simulink model "single_camera_xy_tracking_base_kf_fixed"  (R2025b)
settings: Solver=FixedStepDiscrete  StartTime=0  StopTime=T_end  FixedStep=Ts  RelTol=1e-3
InitFcn:
  | % 获取当前.slx模型所在文件夹
  | model_path = fileparts(which(gcs));
  | % 向上跳转、拼接目标函数所在文件夹（根据你的目录调整）
  | func_folder = fullfile(model_path,'..', 'config');
  | % 添加到搜索路径
  | addpath(func_folder);
  | % 执行初始化函数
  | init_single_camera_xy_tracking;
values from neighbouring files (symbols this model uses):
  a_xy_max = 2.0    (= 2)    [init_single_camera_xy_tracking.m]    (also in init_single_camera_xy_tracking_5dof.m; init_single_camera_xy_tracking_base_cv_kf.m; init_single_camera_xy_tracking_cv_ekf.m)
  adapt_max = 0.0    (= 0)    [init_single_camera_xy_tracking.m]    (also in init_single_camera_xy_tracking_5dof.m)
  camera_velocity_feedback_timeout_sec = 0.5    [init_single_camera_xy_tracking.m]    (also in init_single_camera_xy_tracking_5dof.m)
  controller_enable = true    [init_single_camera_xy_tracking.m]    (also in init_single_camera_xy_tracking_5dof.m; init_single_camera_xy_tracking_base_cv_kf.m; init_single_camera_xy_tracking_cv_ekf.m)
  cx = 1000    [init_single_camera_xy_tracking.m]    (also in init_single_camera_xy_tracking_5dof.m; init_single_camera_xy_tracking_base_cv_kf.m; init_single_camera_xy_tracking_cv_ekf.m)
  cy = 592    [init_single_camera_xy_tracking.m]    (also in init_single_camera_xy_tracking_5dof.m; init_single_camera_xy_tracking_base_cv_kf.m; init_single_camera_xy_tracking_cv_ekf.m)
  ekf_gate_threshold = 5.991    [init_single_camera_xy_tracking.m]    (also in init_single_camera_xy_tracking_5dof.m; init_single_camera_xy_tracking_cv_ekf.m)
  ekf_reset_timeout_sec = 0.50    (= 0.5)    [init_single_camera_xy_tracking.m]    (also in init_single_camera_xy_tracking_5dof.m; init_single_camera_xy_tracking_cv_ekf.m)
  enable_adaptation = false    [init_single_camera_xy_tracking_5dof.m]
  enable_ekf_feedforward = true    [init_single_camera_xy_tracking.m]    (also in init_single_camera_xy_tracking_5dof.m; init_single_camera_xy_tracking_base_cv_kf.m; init_single_camera_xy_tracking_cv_ekf.m)
  enable_proportional = true    [init_single_camera_xy_tracking.m]    (also in init_single_camera_xy_tracking_5dof.m; init_single_camera_xy_tracking_base_cv_kf.m; init_single_camera_xy_tracking_cv_ekf.m)
  fx = 2057    [init_single_camera_xy_tracking.m]    (also in init_single_camera_xy_tracking_5dof.m; init_single_camera_xy_tracking_base_cv_kf.m; init_single_camera_xy_tracking_cv_ekf.m)
  fy = 2054    [init_single_camera_xy_tracking.m]    (also in init_single_camera_xy_tracking_5dof.m; init_single_camera_xy_tracking_base_cv_kf.m; init_single_camera_xy_tracking_cv_ekf.m)
  gamma_adapt = 0.0    (= 0)    [init_single_camera_xy_tracking.m]    (also in init_single_camera_xy_tracking_5dof.m)
  joint_state_timeout_sec = 0.10    (= 0.1)    [init_single_camera_xy_tracking.m]    (also in init_single_camera_xy_tracking_5dof.m; init_single_camera_xy_tracking_base_cv_kf.m; init_single_camera_xy_tracking_cv_ekf.m)
  k_ff = 0.5    [init_single_camera_xy_tracking.m]    (also in init_single_camera_xy_tracking_5dof.m; init_single_camera_xy_tracking_base_cv_kf.m; init_single_camera_xy_tracking_cv_ekf.m)
  Kpx = 1.0    (= 1)    [init_single_camera_xy_tracking.m]    (also in init_single_camera_xy_tracking_5dof.m; init_single_camera_xy_tracking_base_cv_kf.m; init_single_camera_xy_tracking_cv_ekf.m)
  Kpy = 1.0    (= 1)    [init_single_camera_xy_tracking.m]    (also in init_single_camera_xy_tracking_5dof.m; init_single_camera_xy_tracking_base_cv_kf.m; init_single_camera_xy_tracking_cv_ekf.m)
  P0 = diag([0.05^2, 0.05^2, 0.20^2, 0.20^2, 0.50^2, 0.50^2])    [init_single_camera_xy_tracking.m]    (also in init_single_camera_xy_tracking_5dof.m = diag([.05 .05 .2 .2 .5 .5].^2); init_single_camera_xy_tracking_base_cv_kf.m = diag([.05 .05 .20 .20].^2); init_single_camera_xy_tracking_cv_ekf.m = diag([.05 .05 .20 .20].^2))
  Q_ekf = diag([1e-12, 1e-12, 1e-12, 1e-12, 1e-4, 1e-4])    [init_single_camera_xy_tracking.m]    (also in init_single_camera_xy_tracking_5dof.m = diag([1e-12 1e-12 1e-12 1e-12 1e-4 1e-4]); init_single_camera_xy_tracking_cv_ekf.m = sigma_acc_cv^2*[      Ts^4/4 0 Ts^3/2 0;      0 Ts^4/4 0 Ts^)
  R_ekf = diag([1e-8, 1e-8])    [init_single_camera_xy_tracking.m]    (also in init_single_camera_xy_tracking_5dof.m = diag([1e-8 1e-8]); init_single_camera_xy_tracking_cv_ekf.m = diag([1e-8 1e-8]))
  sigma_adapt = 0.0    (= 0)    [init_single_camera_xy_tracking.m]    (also in init_single_camera_xy_tracking_5dof.m)
  target_timeout_sec = 0.20    (= 0.2)    [init_single_camera_xy_tracking.m]    (also in init_single_camera_xy_tracking_5dof.m; init_single_camera_xy_tracking_base_cv_kf.m; init_single_camera_xy_tracking_cv_ekf.m)
  Ts = 0.01    [init_single_camera_xy_tracking.m]    (also in init_single_camera_xy_tracking_5dof.m; init_single_camera_xy_tracking_base_cv_kf.m; init_single_camera_xy_tracking_cv_ekf.m)
  v_xy_max = 2.0    (= 2)    [init_single_camera_xy_tracking.m]    (also in init_single_camera_xy_tracking_5dof.m; init_single_camera_xy_tracking_base_cv_kf.m; init_single_camera_xy_tracking_cv_ekf.m)
  Z_hat = 1    [init_single_camera_xy_tracking.m]    (also in init_single_camera_xy_tracking_5dof.m; init_single_camera_xy_tracking_base_cv_kf.m; init_single_camera_xy_tracking_cv_ekf.m)
undefined symbols (not defined in the file or in its folder): data, data_SL_Info
libraries: ros2lib x4, robotmaniplib x3
Description:
  | Fixed-focus monocular XY target tracking. Outputs camera-frame [vx vy 0 0 0 0]; robot kinematics remain external.
settings Model: Creator=ASUS  LastModifiedBy=harry
settings DataIOCC: SignalLogging=off

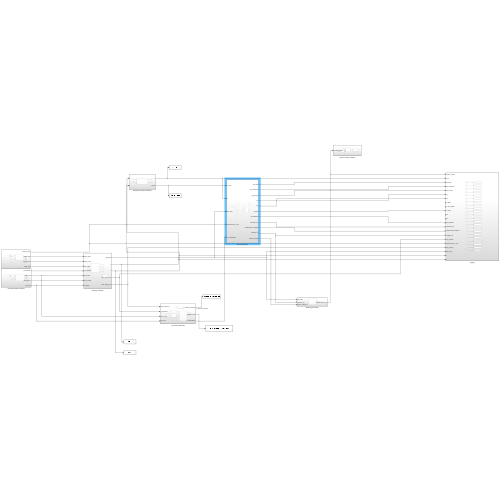
[thumbnail: Simulink's stored preview of the top-level diagram]
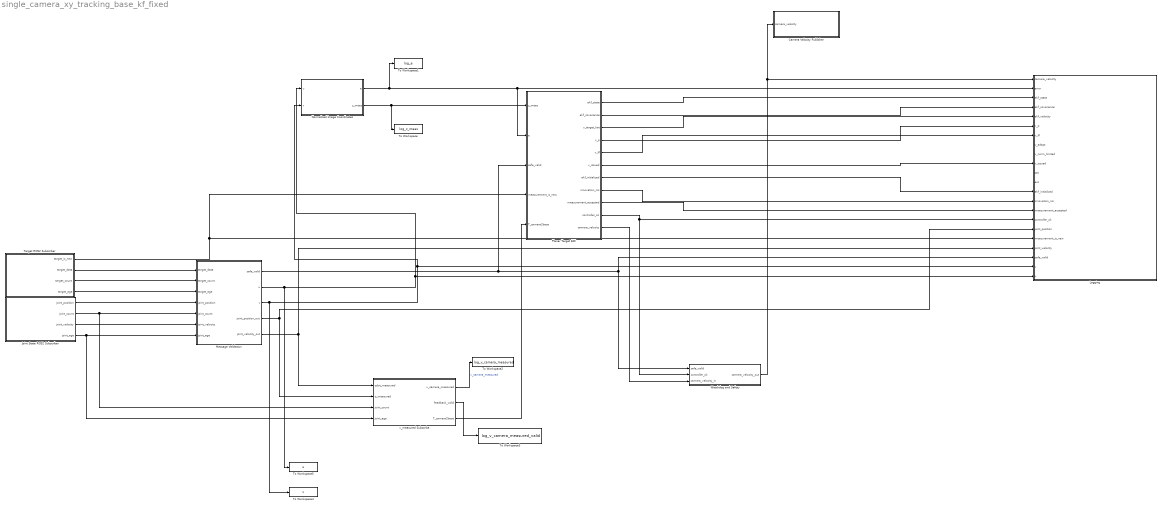
== system single_camera_xy_tracking_base_kf_fixed ==
  Camera Velocity Publisher : Subsystem
  Joint State ROS2 Subscriber : Subsystem
  Logging : Subsystem
  Message Validation : Subsystem
  Normalized Image Coordinates : Subsystem
  Planar Target EKF : Subsystem
  Target ROS2 Subscriber : Subsystem
  To Workspace : ToWorkspace  VariableName=log_z_meas  SaveFormat=Timeseries  SampleTime=-1
  To Workspace1 : ToWorkspace  VariableName=log_e  SaveFormat=Timeseries  SampleTime=-1
  To Workspace2 : ToWorkspace  VariableName=log_v_camera_measured  SaveFormat=Timeseries  SampleTime=-1
  To Workspace3 : ToWorkspace  VariableName=log_v_camera_measured_valid  SaveFormat=Timeseries  SampleTime=-1
  To Workspace4 : ToWorkspace  VariableName=v  SaveFormat=Timeseries  SampleTime=-1
  To Workspace5 : ToWorkspace  VariableName=u  SaveFormat=Timeseries  SampleTime=-1
  Watchdog and Safety : Subsystem
  v_measured Subscribe : Subsystem
  wires:
  Target ROS2 Subscriber/4(target_age) -> Message Validation/3(target_age)
  Target ROS2 Subscriber/2(target_data) -> Message Validation/1(target_data)
  Target ROS2 Subscriber/3(target_count) -> Message Validation/2(target_count)
  Planar Target EKF/3(v_target_hat) -> Logging/5(ekf_velocity)
  Message Validation/2(u) -> Normalized Image Coordinates/1(u), Logging/22(u), To Workspace5/1
  Planar Target EKF/10(controller_ok) -> Watchdog and Safety/2(controller_ok), Logging/16(controller_ok)
  Joint State ROS2 Subscriber/4(joint_age) -> v_measured Subscribe/4(joint_age), Message Validation/7(joint_age)
  Joint State ROS2 Subscriber/2(joint_count) -> v_measured Subscribe/3(joint_count), Message Validation/5(joint_count)
  Joint State ROS2 Subscriber/1(joint_position) -> Message Validation/4(joint_position)
  Joint State ROS2 Subscriber/3(joint_velocity) -> Message Validation/6(joint_velocity)
  Message Validation/1(safe_valid) -> Logging/20(safe_valid), Watchdog and Safety/1(safe_valid), Planar Target EKF/3(safe_valid)
  Message Validation/3(v) -> To Workspace4/1, Normalized Image Coordinates/2(v), Logging/21(v)
  Message Validation/4(joint_position_out) -> v_measured Subscribe/2(q_measured), Logging/17(joint_position)
  Message Validation/5(joint_velocity_out) -> v_measured Subscribe/1(qdot_measured), Logging/19(joint_velocity)
  Normalized Image Coordinates/1(e) -> To Workspace1/1, Logging/2(error), Planar Target EKF/2(e)
  Normalized Image Coordinates/2(z_meas) -> To Workspace/1, Planar Target EKF/1(z_meas)
  Planar Target EKF/1(ekf_state) -> Logging/3(ekf_state)
  Planar Target EKF/2(ekf_covariance) -> Logging/4(ekf_covariance)
  Planar Target EKF/9(measurement_accepted) -> Logging/15(measurement_accepted)
  Planar Target EKF/7(ekf_initialized) -> Logging/13(ekf_initialized)
  Planar Target EKF/8(innovation_nis) -> Logging/14(innovation_nis)
  Planar Target EKF/4(v_p) -> Logging/6(v_p)
  Planar Target EKF/5(v_ff) -> Logging/7(v_ff)
  Planar Target EKF/6(v_issued) -> Logging/10(v_issued)
  Planar Target EKF/11(camera_velocity) -> Watchdog and Safety/3(camera_velocity_in)
  Watchdog and Safety/1(camera_velocity_out) -> Camera Velocity Publisher/1(camera_velocity), Logging/1(camera_velocity)
  Target ROS2 Subscriber/1(target_is_new) -> Planar Target EKF/4(measurement_is_new), Logging/18(measurement_is_new)
  v_measured Subscribe/1(v_camera_measured) -> To Workspace2/1  "v_camera_measured"
  v_measured Subscribe/2(feedback_valid) -> To Workspace3/1
  v_measured Subscribe/3(T_camera2base) -> Planar Target EKF/5(T_camera2base)

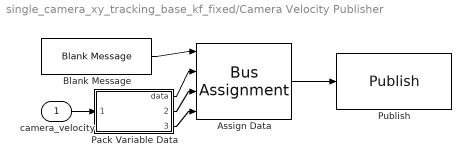
== system single_camera_xy_tracking_base_kf_fixed/Camera Velocity Publisher ==
  camera_velocity : Inport
  Assign Data : BusAssignment  AssignedSignals=data,data_SL_Info.CurrentLength,data_SL_Info.ReceivedLength
  Blank Message : ros2lib/Blank Message  messageClass=Message  entityType=std_msgs/Float64MultiArray  messageType=std_msgs/Float64MultiArray  SampleTime=Ts
  Pack Variable Data : MATLAB Function  TreatAsAtomicUnit=on
  Publish : ros2lib/Publish  topicSource=Select from ROS network  topic=/simulink/camera_velocity  messageType=std_msgs/Float64MultiArray  QOSHistory=Keep last  QOSDepth=1  QOSReliability=Reliable  QOSDurability=Volatile  QOSDeadline=Inf  QOSLifespan=Inf  QOSLiveliness=Automatic  QOSLeaseDuration=Inf  QOSAvoidROSNamespaceConventions=off
  wires:
  Blank Message/1 -> Assign Data/1
  Assign Data/1 -> Publish/1
  camera_velocity/1 -> Pack Variable Data/1(camera_velocity)
  Pack Variable Data/1(data) -> Assign Data/2
  Pack Variable Data/2(current_length) -> Assign Data/3
  Pack Variable Data/3(received_length) -> Assign Data/4

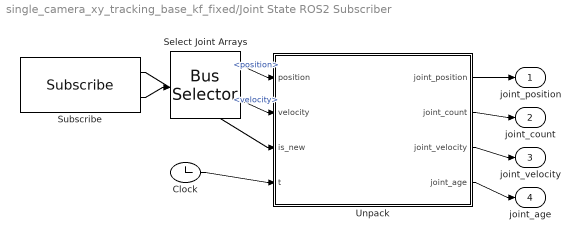
== system single_camera_xy_tracking_base_kf_fixed/Joint State ROS2 Subscriber ==
  Clock : Clock
  Select Joint Arrays : BusSelector  OutputSignals=position,velocity
  Subscribe : ros2lib/Subscribe  topicSource=Select from ROS network  topic=/franka/joint_states  messageType=sensor_msgs/JointState  sampleTime=Ts  QOSHistory=Keep last  QOSDepth=1  QOSReliability=Best effort  QOSDurability=Volatile  QOSDeadline=Inf  QOSLifespan=Inf  QOSLiveliness=Automatic  QOSLeaseDuration=Inf  QOSAvoidROSNamespaceConventions=off
  Unpack : MATLAB Function  TreatAsAtomicUnit=on
  joint_position : Outport
  joint_count : Outport  Port=2
  joint_velocity : Outport  Port=3
  joint_age : Outport  Port=4
  wires:
  Unpack/1(joint_position) -> joint_position/1
  Unpack/2(joint_count) -> joint_count/1
  Unpack/3(joint_velocity) -> joint_velocity/1
  Unpack/4(joint_age) -> joint_age/1
  Select Joint Arrays/1 -> Unpack/1(position)  "<position>"
  Select Joint Arrays/2 -> Unpack/2(velocity)  "<velocity>"
  Clock/1 -> Unpack/4(t)
  Subscribe/2 -> Select Joint Arrays/1
  Subscribe/1 -> Unpack/3(is_new)

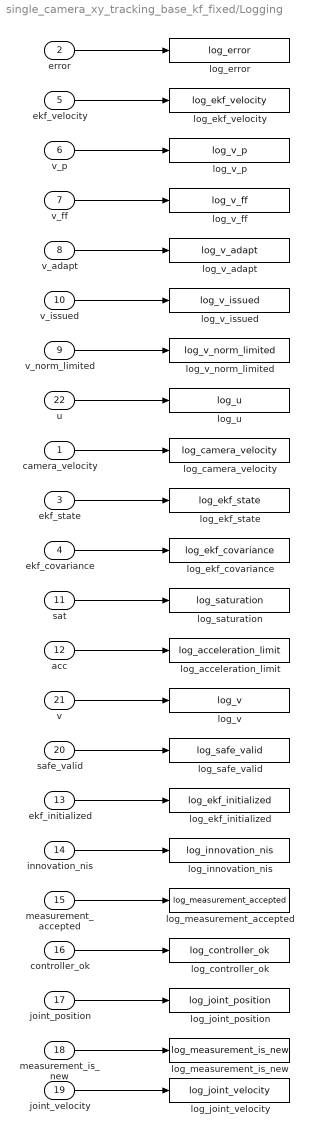
== system single_camera_xy_tracking_base_kf_fixed/Logging ==
  camera_velocity : Inport
  error : Inport  Port=2
  ekf_state : Inport  Port=3
  ekf_covariance : Inport  Port=4
  ekf_velocity : Inport  Port=5
  v_p : Inport  Port=6
  v_ff : Inport  Port=7
  v_adapt : Inport  Port=8
  v_norm_limited : Inport  Port=9
  v_issued : Inport  Port=10
  sat : Inport  Port=11
  acc : Inport  Port=12
  ekf_initialized : Inport  Port=13
  innovation_nis : Inport  Port=14
  measurement_accepted : Inport  Port=15
  controller_ok : Inport  Port=16
  joint_position : Inport  Port=17
  measurement_is_new : Inport  Port=18
  joint_velocity : Inport  Port=19
  safe_valid : Inport  Port=20
  v : Inport  Port=21
  u : Inport  Port=22
  log_acceleration_limit : ToWorkspace  VariableName=log_acceleration_limit  SaveFormat=Structure With Time  SampleTime=-1
  log_camera_velocity : ToWorkspace  VariableName=log_camera_velocity  SaveFormat=Structure With Time  SampleTime=-1
  log_controller_ok : ToWorkspace  VariableName=log_controller_ok  SaveFormat=Structure With Time  SampleTime=-1
  log_ekf_covariance : ToWorkspace  VariableName=log_ekf_covariance  SaveFormat=Structure With Time  SampleTime=-1
  log_ekf_initialized : ToWorkspace  VariableName=log_ekf_initialized  SaveFormat=Structure With Time  SampleTime=-1
  log_ekf_state : ToWorkspace  VariableName=log_ekf_state  SaveFormat=Structure With Time  SampleTime=-1
  log_ekf_velocity : ToWorkspace  VariableName=log_ekf_velocity  SaveFormat=Structure With Time  SampleTime=-1
  log_error : ToWorkspace  VariableName=log_error  SaveFormat=Structure With Time  SampleTime=-1
  log_innovation_nis : ToWorkspace  VariableName=log_innovation_nis  SaveFormat=Structure With Time  SampleTime=-1
  log_joint_position : ToWorkspace  VariableName=log_joint_position  SaveFormat=Structure With Time  SampleTime=-1
  log_joint_velocity : ToWorkspace  VariableName=log_joint_velocity  SaveFormat=Structure With Time  SampleTime=-1
  log_measurement_accepted : ToWorkspace  VariableName=log_measurement_accepted  SaveFormat=Structure With Time  SampleTime=-1
  log_measurement_is_new : ToWorkspace  VariableName=log_measurement_is_new  SaveFormat=Structure With Time  SampleTime=-1
  log_safe_valid : ToWorkspace  VariableName=log_safe_valid  SaveFormat=Structure With Time  SampleTime=-1
  log_saturation : ToWorkspace  VariableName=log_saturation  SaveFormat=Structure With Time  SampleTime=-1
  log_u : ToWorkspace  VariableName=log_u  SaveFormat=Structure With Time  SampleTime=-1
  log_v : ToWorkspace  VariableName=log_v  SaveFormat=Structure With Time  SampleTime=-1
  log_v_adapt : ToWorkspace  VariableName=log_v_adapt  SaveFormat=Structure With Time  SampleTime=-1
  log_v_ff : ToWorkspace  VariableName=log_v_ff  SaveFormat=Structure With Time  SampleTime=-1
  log_v_issued : ToWorkspace  VariableName=log_v_issued  SaveFormat=Structure With Time  SampleTime=-1
  log_v_norm_limited : ToWorkspace  VariableName=log_v_norm_limited  SaveFormat=Structure With Time  SampleTime=-1
  log_v_p : ToWorkspace  VariableName=log_v_p  SaveFormat=Structure With Time  SampleTime=-1
  wires:
  error/1 -> log_error/1
  ekf_velocity/1 -> log_ekf_velocity/1
  v_p/1 -> log_v_p/1
  v_ff/1 -> log_v_ff/1
  v_adapt/1 -> log_v_adapt/1
  v_issued/1 -> log_v_issued/1
  u/1 -> log_u/1
  camera_velocity/1 -> log_camera_velocity/1
  ekf_state/1 -> log_ekf_state/1
  ekf_covariance/1 -> log_ekf_covariance/1
  sat/1 -> log_saturation/1
  acc/1 -> log_acceleration_limit/1
  v/1 -> log_v/1
  safe_valid/1 -> log_safe_valid/1
  ekf_initialized/1 -> log_ekf_initialized/1
  innovation_nis/1 -> log_innovation_nis/1
  measurement_accepted/1 -> log_measurement_accepted/1
  controller_ok/1 -> log_controller_ok/1
  joint_position/1 -> log_joint_position/1
  joint_velocity/1 -> log_joint_velocity/1
  measurement_is_new/1 -> log_measurement_is_new/1
  v_norm_limited/1 -> log_v_norm_limited/1

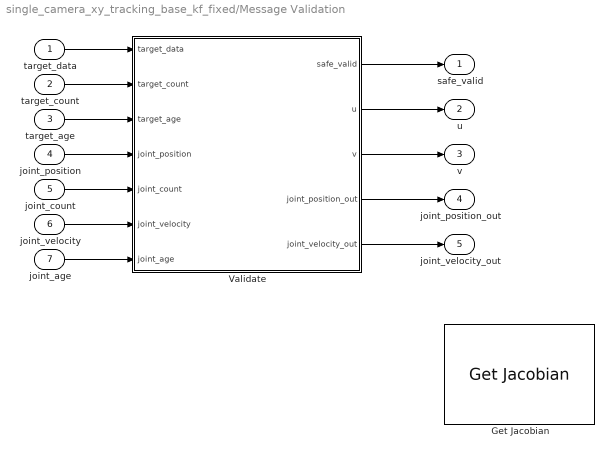
== system single_camera_xy_tracking_base_kf_fixed/Message Validation ==
  target_data : Inport
  target_count : Inport  Port=2
  target_age : Inport  Port=3
  joint_position : Inport  Port=4
  joint_count : Inport  Port=5
  joint_velocity : Inport  Port=6
  joint_age : Inport  Port=7
  Get Jacobian : robotmaniplib/Get Jacobian  RigidBodyTree=twoJointRigidBodyTree  EndEffector=tool  SimulateUsing=Interpreted execution
  Validate : MATLAB Function  TreatAsAtomicUnit=on
  safe_valid : Outport
  u : Outport  Port=2
  v : Outport  Port=3
  joint_position_out : Outport  Port=4
  joint_velocity_out : Outport  Port=5
  wires:
  Validate/1(safe_valid) -> safe_valid/1
  Validate/2(u) -> u/1
  Validate/3(v) -> v/1
  Validate/4(joint_position_out) -> joint_position_out/1
  Validate/5(joint_velocity_out) -> joint_velocity_out/1
  target_data/1 -> Validate/1(target_data)
  target_count/1 -> Validate/2(target_count)
  target_age/1 -> Validate/3(target_age)
  joint_position/1 -> Validate/4(joint_position)
  joint_count/1 -> Validate/5(joint_count)
  joint_velocity/1 -> Validate/6(joint_velocity)
  joint_age/1 -> Validate/7(joint_age)

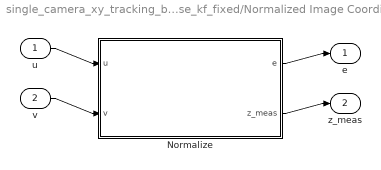
== system single_camera_xy_tracking_base_kf_fixed/Normalized Image Coordinates ==
  u : Inport
  v : Inport  Port=2
  Normalize : MATLAB Function  TreatAsAtomicUnit=on
  e : Outport
  z_meas : Outport  Port=2
  wires:
  u/1 -> Normalize/1(u)
  v/1 -> Normalize/2(v)
  Normalize/1(e) -> e/1
  Normalize/2(z_meas) -> z_meas/1

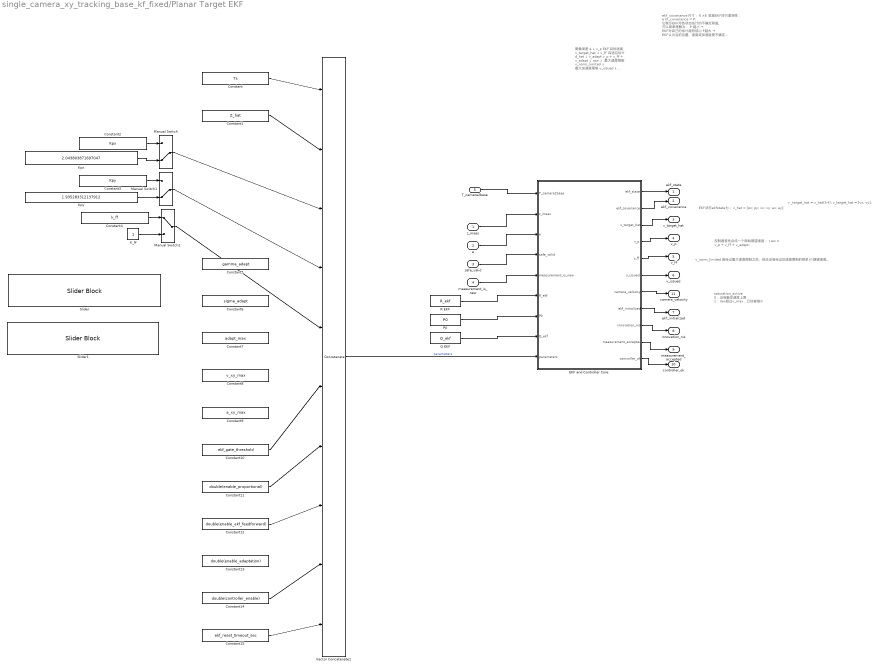
== system single_camera_xy_tracking_base_kf_fixed/Planar Target EKF ==
  note: saturation_active
      | 0：没有触发速度上限
      | 1：raw超过v_max，已经被缩小
  note: ekf_covariance
      | 尺寸：
      | 6 ×6
      | 就是EKF协方差矩阵：
      | e kf_covariance = P;
      | 它表示EKF对各状态估计的不确定程度。
      | 可以简单理解为：
      | P 越小
      | → EKF对自己的估计越有信心
      |
      | P越大
      | → EKF认为当前位置、速度或加速度更不确定
      | 重点可以观察：
      | d iag(P)
      | 也就是：
      | 位 置方差
      | 速度方差
      | 加速度方差
  note: 图像误差 e
      |     ↓
      | v_p
      |
      | EKF目标速度 v_target_hat
      |     ↓
      | v_ff
      |
      | 自适应估计 d_hat
      |     ↓
      | v_adapt
      |
      | v_p + v_ff + v_adapt
      |     ↓
      | raw
      |     ↓ 最大速度限制
      | v_norm_limited
      |     ↓ 最大加速度限制
      | v_issued
      |     ↓ 扩展为6维
      | camera_velocity
  note: EKF状态ekfstate为： x_hat = [px; py; vx; vy; ax; ay];
  note: v _target_hat = x_hat(3:4); v_target_hat = [vx; vy];
  note: 控制器首先合成一个原始期望速度：
      | r aw = v_p + v_ff + v_adapt;
  note: v_norm_limited 是经过最大速度限制之后、但还没有经过加速度限制的相机XY期望速度。
  z_meas : Inport
  e : Inport  Port=2
  safe_valid : Inport  Port=3
  measurement_is_new : Inport  Port=4
  T_camera2base : Inport  Port=5
  Constant : Constant  Value=Ts
  Constant1 : Constant  Value=Z_hat
  Constant10 : Constant  Value=ekf_gate_threshold
  Constant11 : Constant  Value=double(enable_proportional)
  Constant12 : Constant  Value=double(enable_ekf_feedforward)
  Constant13 : Constant  Value=double(enable_adaptation)
  Constant14 : Constant  Value=double(controller_enable)
  Constant15 : Constant  Value=ekf_reset_timeout_sec
  Constant2 : Constant  Value=Kpx
  Constant3 : Constant  Value=Kpy
  Constant4 : Constant  Value=k_ff
  Constant5 : Constant  Value=gamma_adapt
  Constant6 : Constant  Value=sigma_adapt
  Constant7 : Constant  Value=adapt_max
  Constant8 : Constant  Value=v_xy_max
  Constant9 : Constant  Value=a_xy_max
  EKF and Controller Core : MATLAB Function  TreatAsAtomicUnit=on
  K_ff : Constant
  Kpx : Constant  Value=2.043803871697047
  Kpy : Constant  Value=1.935283312137912
  Manual Switch : ManualSwitch  CurrentSetting=0
  Manual Switch1 : ManualSwitch  CurrentSetting=0
  Manual Switch2 : ManualSwitch
  P0 : Constant  Value=P0
  Q EKF : Constant  Value=Q_ekf
  R EKF : Constant  Value=R_ekf
  Slider : SliderBlock  ScaleMax=10
  Slider1 : SliderBlock  ScaleMax=10
  Vector Concatenate1 : Concatenate  NumInputs=10
  ekf_state : Outport
  ekf_covariance : Outport  Port=2
  v_target_hat : Outport  Port=3
  v_p : Outport  Port=4
  v_ff : Outport  Port=5
  v_issued : Outport  Port=6
  ekf_initialized : Outport  Port=7
  innovation_nis : Outport  Port=8
  measurement_accepted : Outport  Port=9
  controller_ok : Outport  Port=10
  camera_velocity : Outport  Port=11
  wires:
  EKF and Controller Core/1(ekf_state) -> ekf_state/1
  EKF and Controller Core/2(ekf_covariance) -> ekf_covariance/1
  EKF and Controller Core/3(v_target_hat) -> v_target_hat/1
  EKF and Controller Core/4(v_p) -> v_p/1
  EKF and Controller Core/5(v_ff) -> v_ff/1
  EKF and Controller Core/6(v_issued) -> v_issued/1
  EKF and Controller Core/7(camera_velocity) -> camera_velocity/1
  EKF and Controller Core/8(ekf_initialized) -> ekf_initialized/1
  EKF and Controller Core/9(innovation_nis) -> innovation_nis/1
  EKF and Controller Core/10(measurement_accepted) -> measurement_accepted/1
  EKF and Controller Core/11(controller_ok) -> controller_ok/1
  z_meas/1 -> EKF and Controller Core/2(z_meas)
  e/1 -> EKF and Controller Core/3(e)
  safe_valid/1 -> EKF and Controller Core/4(safe_valid)
  measurement_is_new/1 -> EKF and Controller Core/5(measurement_is_new)
  Vector Concatenate1/1 -> EKF and Controller Core/9(parameters)  "parameters"
  P0/1 -> EKF and Controller Core/7(P0)
  Q EKF/1 -> EKF and Controller Core/8(Q_ekf)
  R EKF/1 -> EKF and Controller Core/6(R_ekf)
  Constant/1 -> Vector Concatenate1/1
  Constant1/1 -> Vector Concatenate1/2
  Constant10/1 -> Vector Concatenate1/6
  Constant11/1 -> Vector Concatenate1/7
  Constant12/1 -> Vector Concatenate1/8
  Constant14/1 -> Vector Concatenate1/9
  Constant15/1 -> Vector Concatenate1/10
  T_camera2base/1 -> EKF and Controller Core/1(T_camera2base)
  Constant2/1 -> Manual Switch/1
  Manual Switch/1 -> Vector Concatenate1/3
  Kpx/1 -> Manual Switch/2
  Kpy/1 -> Manual Switch1/2
  Constant3/1 -> Manual Switch1/1
  Manual Switch1/1 -> Vector Concatenate1/4
  Constant4/1 -> Manual Switch2/1
  Manual Switch2/1 -> Vector Concatenate1/5
  K_ff/1 -> Manual Switch2/2

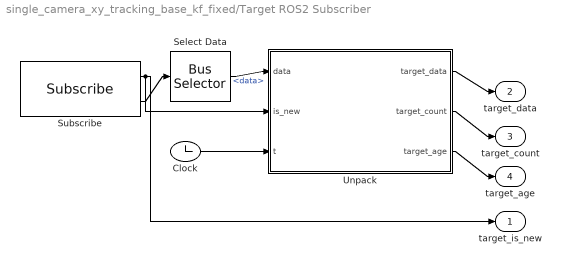
== system single_camera_xy_tracking_base_kf_fixed/Target ROS2 Subscriber ==
  Clock : Clock
  Select Data : BusSelector  OutputSignals=data
  Subscribe : ros2lib/Subscribe  topicSource=Select from ROS network  topic=/apriltag_detector/target_position  messageType=std_msgs/Float64MultiArray  sampleTime=Ts  QOSHistory=Keep last  QOSDepth=1  QOSReliability=Best effort  QOSDurability=Volatile  QOSDeadline=Inf  QOSLifespan=Inf  QOSLiveliness=Automatic  QOSLeaseDuration=Inf  QOSAvoidROSNamespaceConventions=off
  Unpack : MATLAB Function  TreatAsAtomicUnit=on
  target_is_new : Outport
  target_data : Outport  Port=2
  target_count : Outport  Port=3
  target_age : Outport  Port=4
  wires:
  Unpack/1(target_data) -> target_data/1
  Unpack/2(target_count) -> target_count/1
  Unpack/3(target_age) -> target_age/1
  Select Data/1 -> Unpack/1(data)  "<data>"
  Clock/1 -> Unpack/3(t)
  Subscribe/2 -> Select Data/1
  Subscribe/1 -> Unpack/2(is_new), target_is_new/1

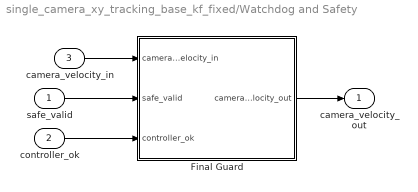
== system single_camera_xy_tracking_base_kf_fixed/Watchdog and Safety ==
  safe_valid : Inport
  controller_ok : Inport  Port=2
  camera_velocity_in : Inport  Port=3
  Final Guard : MATLAB Function  TreatAsAtomicUnit=on
  camera_velocity_out : Outport
  wires:
  camera_velocity_in/1 -> Final Guard/1(camera_velocity_in)
  safe_valid/1 -> Final Guard/2(safe_valid)
  controller_ok/1 -> Final Guard/3(controller_ok)
  Final Guard/1(camera_velocity_out) -> camera_velocity_out/1

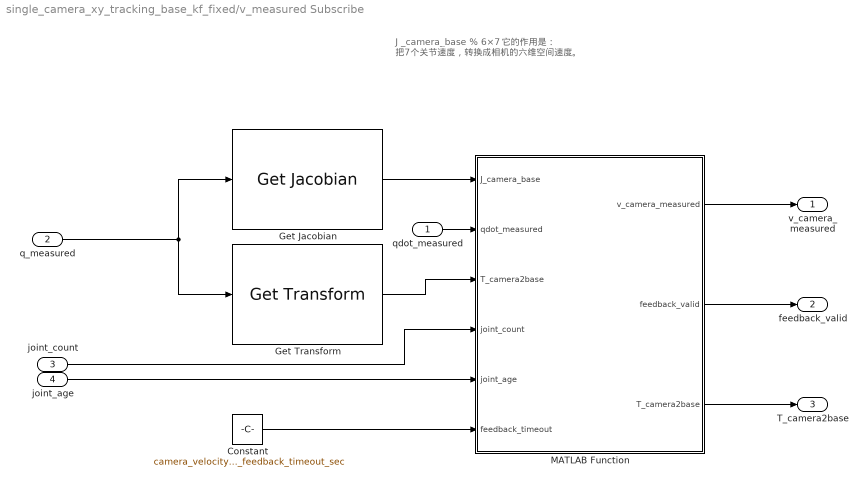
== system single_camera_xy_tracking_base_kf_fixed/v_measured Subscribe ==
  note: J _camera_base % 6×7
      | 它的作用是：
      | 把7个关节速度，转换成相机的六维空间速度。
  qdot_measured : Inport
  q_measured : Inport  Port=2
  joint_count : Inport  Port=3
  joint_age : Inport  Port=4
  Constant : Constant  Value=camera_velocity_feedback_timeout_sec
  Get Jacobian : robotmaniplib/Get Jacobian  RigidBodyTree=fr3_camera_robot  EndEffector=camera_link  SimulateUsing=Interpreted execution
  Get Transform : robotmaniplib/Get Transform  RigidBodyTree=fr3_camera_robot  SourceBody=camera_link  TargetBody=base  SimulateUsing=Interpreted execution
  MATLAB Function : MATLAB Function  TreatAsAtomicUnit=on
  v_camera_measured : Outport
  feedback_valid : Outport  Port=2
  T_camera2base : Outport  Port=3
  wires:
  q_measured/1 -> Get Transform/1, Get Jacobian/1
  qdot_measured/1 -> MATLAB Function/2(qdot_measured)
  Get Jacobian/1 -> MATLAB Function/1(J_camera_base)
  Get Transform/1 -> MATLAB Function/3("T_camera2base ")
  joint_count/1 -> MATLAB Function/4(joint_count)
  joint_age/1 -> MATLAB Function/5(joint_age)
  Constant/1 -> MATLAB Function/6(feedback_timeout)
  MATLAB Function/1(v_camera_measured) -> v_camera_measured/1
  MATLAB Function/2(feedback_valid) -> feedback_valid/1
  MATLAB Function/3(T_camera2base) -> T_camera2base/1

== matlab function single_camera_xy_tracking_base_kf_fixed/Planar Target EKF/EKF and Controller Core ==
  data: T_camera2base input; z_meas input size=[2 1]; ekf_state output size=[6 1]; e input size=[2 1]; safe_valid input size=1; measurement_is_new input; R_ekf input size=[2 2]; P0 input size=[6 6]; Q_ekf input size=[6 6]; parameters input size=[16 1]; ekf_covariance output size=[6 6]; v_target_hat output size=[2 1]; v_p output size=[2 1]; v_ff output size=[2 1]; v_issued output size=[2 1]; camera_velocity output size=[6 1]; ekf_initialized output size=1; innovation_nis output size=1; measurement_accepted output size=1; controller_ok output size=1
function [ ...
    ekf_state, ...
    ekf_covariance, ...
    v_target_hat, ...
    v_p, ...
    v_ff, ...
    v_issued, ...
    camera_velocity, ...
    ekf_initialized, ...
    innovation_nis, ...
    measurement_accepted, ...
    controller_ok] = fcn( ...
    T_camera2base, ...
    z_meas, ...
    e, ...
    safe_valid, ...
    measurement_is_new, ...
    R_ekf, ...
    P0, ...
    Q_ekf, ...
    parameters)
%#codegen
%
% Base坐标系目标状态估计与相机XY速度控制器。
%
% ==================== 坐标系定义 ====================
%
% KF状态全部在机器人Base坐标系中：
%
% x_hat = [X_B; Y_B; Vx_B; Vy_B; Ax_B; Ay_B]
%
% z_meas为相机坐标系中的目标XY位置：
%
% z_meas = [X_C; Y_C]
%
% 根据固定深度Z_hat构造目标相机系三维位置：
%
% p_target_C = [X_C; Y_C; Z_hat]
%
% 再通过T_camera2base转换到机器人Base坐标系：
%
% p_target_B = R_BC*p_target_C + t_BC
%
% 控制器输出仍在相机坐标系：
%
% camera_velocity = [vx_C; vy_C; 0; 0; 0; 0]
%
% ==================== 输入矩阵要求 ====================
%
% T_camera2base：4×4，相机坐标系到Base坐标系的变换
%
%   p_B = T_camera2base*[p_C;1]
%
% R_ekf：2×2，相机系XY位置测量噪声协方差
% P0：6×6，Base系状态初始协方差
% Q_ekf：6×6，Base系过程噪声协方差
%
% ==================== parameters ====================
%
% parameters(1)  = Ts
% parameters(2)  = Z_hat
% parameters(3)  = Kpx
% parameters(4)  = Kpy
% parameters(5)  = k_ff
% parameters(6)  = NIS gate
% parameters(7)  = enable_p
% parameters(8)  = enable_ff
% parameters(9)  = controller_enable
% parameters(10) = reset_timeout


%% 1. 持久状态

persistent x_hat
persistent P
persistent e_hold
persistent invalid_time
persistent initialized


%% 2. 初始化

if isempty(initialized)

    x_hat = zeros(6,1);
    P = P0;

    e_hold = zeros(2,1);

    invalid_time = 0.0;
    initialized = false;
end


%% 3. 参数解析

Ts = parameters(1);
Z_hat = parameters(2);

Kpx = parameters(3);
Kpy = parameters(4);

k_ff = parameters(5);
gate = parameters(6);

enable_p = parameters(7) > 0.5;
enable_ff = parameters(8) > 0.5;

controller_enable = parameters(9) > 0.5;
reset_timeout = parameters(10);

safe_valid = safe_valid > 0.5;
measurement_is_new = measurement_is_new > 0.5;


%% 4. 默认输出

ekf_state = x_hat;
ekf_covariance = P;

% Base坐标系中的目标XY速度。
v_target_hat = zeros(2,1);

% 以下控制速度均在相机坐标系。
v_p = zeros(2,1);
v_ff = zeros(2,1);
v_issued = zeros(2,1);

camera_velocity = zeros(6,1);

ekf_initialized = initialized;

innovation_nis = NaN;
measurement_accepted = false;
controller_ok = false;


%% 5. 状态模型

% Base坐标系恒加速度模型：
%
% X(k+1)  = X(k)  + Ts*Vx(k) + 0.5*Ts^2*Ax(k)
% Y(k+1)  = Y(k)  + Ts*Vy(k) + 0.5*Ts^2*Ay(k)
% Vx(k+1) = Vx(k) + Ts*Ax(k)
% Vy(k+1) = Vy(k) + Ts*Ay(k)

F = [ ...
    1 0 Ts 0  0.5*Ts*Ts 0;
    0 1 0  Ts 0  0.5*Ts*Ts;
    0 0 1  0  Ts 0;
    0 0 0  1  0  Ts;
    0 0 0  0  1  0;
    0 0 0  0  0  1];

% 只测量Base坐标系目标XY位置。
H = [ ...
    1 0 0 0 0 0;
    0 1 0 0 0 0];

I6 = eye(6);


%% 6. 参数检查

parameter_ok = ...
    numel(parameters) >= 10 && ...
    isequal(size(P0),[6 6]) && ...
    isequal(size(Q_ekf),[6 6]) && ...
    isequal(size(R_ekf),[2 2]) && ...
    all(isfinite(parameters(:))) && ...
    all(isfinite(P0(:))) && ...
    all(isfinite(Q_ekf(:))) && ...
    all(isfinite(R_ekf(:))) && ...
    Ts > 0 && ...
    Z_hat > 0 && ...
    gate > 0 && ...
    reset_timeout >= Ts;

if ~parameter_ok

    x_hat = zeros(6,1);
    P = P0;

    e_hold = zeros(2,1);
    invalid_time = 0.0;
    initialized = false;

    ekf_state = x_hat;
    ekf_covariance = P;
    ekf_initialized = false;

    return
end


%% 7. 检查相机位姿

pose_matrix_ok = ...
    isequal(size(T_camera2base),[4 4]) && ...
    all(isfinite(T_camera2base(:)));

R_base_camera = eye(3);
t_base_camera = zeros(3,1);

pose_ok = false;

if pose_matrix_ok

    R_candidate = T_camera2base(1:3,1:3);
    t_candidate = T_camera2base(1:3,4);

    orthogonality_error = ...
        norm(R_candidate'*R_candidate - eye(3),'fro');

    determinant_error = ...
        abs(det(R_candidate) - 1.0);

    last_row_error = ...
        norm(T_camera2base(4,:) - [0 0 0 1]);

    pose_ok = ...
        orthogonality_error < 1e-3 && ...
        determinant_error < 1e-3 && ...
        last_row_error < 1e-6 && ...
        all(isfinite(t_candidate));

    if pose_ok
        R_base_camera = R_candidate;
        t_base_camera = t_candidate;
    end
end


%% 8. 检查视觉输入

vision_signal_ok = ...
    safe_valid && ...
    numel(z_meas) == 2 && ...
    numel(e) == 2 && ...
    all(isfinite(z_meas(:))) && ...
    all(isfinite(e(:)));


%% 9. 输入无效处理

if ~vision_signal_ok

    % 已初始化时继续执行纯预测。
    if initialized

        x_hat = F*x_hat;

        P = F*P*F' + Q_ekf;
        P = 0.5*(P + P');
    end

    invalid_time = invalid_time + Ts;

    % 没有有效目标时不继续使用旧图像误差。
    e_hold = zeros(2,1);

    state_ok = ...
        all(isfinite(x_hat(:))) && ...
        all(isfinite(P(:))) && ...
        all(diag(P) >= 0);

    if invalid_time >= reset_timeout || ~state_ok

        x_hat = zeros(6,1);
        P = P0;

        initialized = false;
    end

    ekf_state = x_hat;
    ekf_covariance = P;

    v_target_hat = x_hat(3:4);
    ekf_initialized = initialized;

    return
end

invalid_time = 0.0;


%% 10. 构造Base坐标系目标位置测量

measurement_available = ...
    measurement_is_new && ...
    pose_ok;

z_base = zeros(2,1);
R_measurement_base = R_ekf;

if measurement_available

    % 目标在相机坐标系中的三维位置。
    p_target_camera = [ ...
        z_meas(1);
        z_meas(2);
        Z_hat];

    % 转换到机器人Base坐标系。
    p_target_base = ...
        R_base_camera*p_target_camera + ...
        t_base_camera;

    % 当前滤波器只使用Base坐标系XY位置。
    z_base = p_target_base(1:2);

    % 将相机系XY测量噪声近似转换到Base系XY。
    %
    % 当前假设Z_hat没有额外测量噪声。
    measurement_rotation = ...
        R_base_camera(1:2,1:2);

    R_measurement_base = ...
        measurement_rotation*R_ekf* ...
        measurement_rotation';

    R_measurement_base = ...
        0.5*(R_measurement_base + ...
        R_measurement_base');

    measurement_available = ...
        all(isfinite(z_base(:))) && ...
        all(isfinite(R_measurement_base(:)));
end


%% 11. 更新最近一次图像误差

% 图像误差直接用于比例反馈。
% 它不受NIS是否接受Base位置测量的影响。

if measurement_is_new
    e_hold = reshape(e,2,1);
end


%% 12. 初始化滤波器

if ~initialized

    if ~measurement_available
        return
    end

    % 初始Base位置由当前目标测量给出。
    % 初始速度和加速度设为零。
    x_hat = [ ...
        z_base(1);
        z_base(2);
        0;
        0;
        0;
        0];

    P = P0;

    initialized = true;
    measurement_accepted = true;


%% 13. 状态预测与测量更新

else

    % 每个控制周期进行状态预测。
    x_pred = F*x_hat;

    P_pred = F*P*F' + Q_ekf;
    P_pred = 0.5*(P_pred + P_pred');

    % 默认采用预测结果。
    x_hat = x_pred;
    P = P_pred;

    if measurement_available

        % Base坐标系位置残差。
        innovation = ...
            z_base - H*x_pred;

        % 创新协方差。
        S = ...
            H*P_pred*H' + ...
            R_measurement_base;

        if all(isfinite(S(:))) && ...
                rcond(S) > 1e-12

            innovation_nis = ...
                innovation'*(S\innovation);

        else

            innovation_nis = inf;
        end

        % 通过NIS门限后进行测量更新。
        if isfinite(innovation_nis) && ...
                innovation_nis <= gate

            % 卡尔曼增益。
            K = ...
                (P_pred*H')/S;

            % 状态更新。
            x_hat = ...
                x_pred + K*innovation;

            % Joseph形式协方差更新。
            A = I6 - K*H;

            P = ...
                A*P_pred*A' + ...
                K*R_measurement_base*K';

            P = 0.5*(P + P');

            measurement_accepted = true;
        end
    end
end


%% 14. 滤波器状态检查

ekf_ok = ...
    all(isfinite(x_hat(:))) && ...
    all(isfinite(P(:))) && ...
    all(diag(P) >= 0) && ...
    norm(P - P','fro') < 1e-6;

if ~ekf_ok

    x_hat = zeros(6,1);
    P = P0;

    e_hold = zeros(2,1);
    invalid_time = 0.0;
    initialized = false;

    ekf_state = x_hat;
    ekf_covariance = P;

    v_target_hat = zeros(2,1);
    ekf_initialized = false;

    return
end


%% 15. 导出Base坐标系估计结果

ekf_state = x_hat;
ekf_covariance = P;

% Base坐标系目标速度：
% [Vx_B; Vy_B]
v_target_hat = x_hat(3:4);

ekf_initialized = initialized;


%% 16. 控制器使能检查

% 关闭控制器不会清空滤波器状态。
% 只是停止输出机器人速度命令。

if ~controller_enable || ...
        ~initialized || ...
        ~pose_ok

    return
end


%% 17. 比例反馈速度

% e为相机坐标系中的归一化图像误差。
% 因此v_p也在相机坐标系中。

if enable_p

    v_p = Z_hat*[ ...
        Kpx*e_hold(1);
        Kpy*e_hold(2)];
end


%% 18. Base目标速度转换到相机坐标系

% 当前滤波器只估计Base系XY速度。
%
% 暂时假设目标在Base系Z方向速度为0。

v_target_base_3d = [ ...
    x_hat(3);
    x_hat(4);
    0];

% 同一个速度从Base系表达转换为相机系表达。
v_target_camera_3d = ...
    R_base_camera'*v_target_base_3d;

v_target_camera_xy = ...
    v_target_camera_3d(1:2);


%% 19. 目标速度前馈

if enable_ff

    v_ff = ...
        k_ff*v_target_camera_xy;
end


%% 20. 合成速度命令

% v_p和v_ff都在相机坐标系中。
v_issued = ...
    v_p + v_ff;


%% 21. 最终检查与输出

controller_ok = ...
    all(isfinite(v_p(:))) && ...
    all(isfinite(v_ff(:))) && ...
    all(isfinite(v_issued(:)));

if controller_ok

    % 相机六维速度命令：
    % [vx_C; vy_C; vz_C; wx_C; wy_C; wz_C]
    camera_velocity = [ ...
        v_issued;
        0;
        0;
        0;
        0];

else

    v_p = zeros(2,1);
    v_ff = zeros(2,1);
    v_issued = zeros(2,1);

    camera_velocity = zeros(6,1);
end

end

== matlab function single_camera_xy_tracking_base_kf_fixed/Watchdog and Safety/Final Guard ==
  data: camera_velocity_in input size=[6 1]; camera_velocity_out output size=[6 1]; safe_valid input size=1; controller_ok input size=1
function camera_velocity_out = fcn(camera_velocity_in,safe_valid,controller_ok)
%#codegen
camera_velocity_out=zeros(6,1);
if safe_valid && controller_ok && all(isfinite(camera_velocity_in(:)))
    camera_velocity_out=camera_velocity_in;
    camera_velocity_out(3:6)=0;
end
end

== matlab function single_camera_xy_tracking_base_kf_fixed/Camera Velocity Publisher/Pack Variable Data ==
  data: camera_velocity input size=[6 1]; data output size=[128 1]; current_length output size=1; received_length output size=1
function [data,current_length,received_length] = fcn(camera_velocity)
%#codegen
data=zeros(128,1); data(1:6)=camera_velocity;
current_length=uint32(6); received_length=uint32(6);
end

== matlab function single_camera_xy_tracking_base_kf_fixed/Target ROS2 Subscriber/Unpack ==
  data: data input; target_data output size=[3 1]; is_new input size=1; t input size=1; target_count output size=1; target_age output size=1
function [target_data,target_count,target_age] = fcn(data,is_new,t)
%#codegen
persistent last_data last_count last_time
if isempty(last_count), last_data=zeros(3,1); last_count=0.0; last_time=-1.0e6; end
if is_new
    n=numel(data); last_data=zeros(3,1);
    if n>=1, last_data(1)=data(1); end
    if n>=2, last_data(2)=data(2); end
    if n>=3, last_data(3)=data(3); end
    last_count=double(n); last_time=t;
end
target_data=last_data; target_count=last_count; target_age=max(0.0,t-last_time);
end

== matlab function single_camera_xy_tracking_base_kf_fixed/v_measured Subscribe/MATLAB Function ==
  data: J_camera_base input; v_camera_measured output; qdot_measured input; T_camera2base input; joint_count input; joint_age input; feedback_timeout input; feedback_valid output; T_camera2base output
function [v_camera_measured,feedback_valid,T_camera2base] = fcn( ...
    J_camera_base, ...
    qdot_measured, ...
    T_camera2base, ...
    joint_count, ...
    joint_age, ...
    feedback_timeout)
%#codegen
% 将机器人实测关节速度转换为相机坐标系XY线速度。

v_camera_measured = zeros(2,1);
feedback_valid = false;

qdot_measured = reshape( ...
    qdot_measured, ...
    7,1);

input_ok = ...
    joint_count >= 7 && ...
    isfinite(joint_age) && ...
    joint_age <= feedback_timeout && ...
    all(isfinite(qdot_measured(:))) && ...
    all(isfinite(J_camera_base(:))) && ...
    all(isfinite(T_camera2base(:))) && ...
    all(size(J_camera_base) == [6 7]) && ...
    all(size(T_camera2base) == [4 4]);

if ~input_ok
    return
end

%% 关节速度转换为基坐标系相机Twist

% Get Jacobian的输出顺序：
% [omega_x;omega_y;omega_z;v_x;v_y;v_z]
camera_twist_base = ...
    J_camera_base*qdot_measured;

% 基坐标系表达的相机线速度。
v_camera_base = ...
    camera_twist_base(4:6);

%% 转换到相机坐标系表达

% T_base_camera将相机坐标转换到基坐标。
R_base_camera = ...
    T_camera2base(1:3,1:3);

% 因此基坐标速度转到相机坐标需要转置。
v_camera_camera = ...
    R_base_camera'*v_camera_base;

v_camera_measured = ...
    v_camera_camera(1:2);

feedback_valid = ...
    all(isfinite(v_camera_measured));

if ~feedback_valid
    v_camera_measured = zeros(2,1);
end

T_camera2base=T_camera2base;

end

== matlab function single_camera_xy_tracking_base_kf_fixed/Joint State ROS2 Subscriber/Unpack ==
  data: position input; joint_position output size=[7 1]; velocity input; is_new input size=1; t input size=1; joint_count output size=1; joint_velocity output size=[7 1]; joint_age output size=1
function [joint_position,joint_count,joint_velocity,joint_age] = fcn(position,velocity,is_new,t)
%#codegen
persistent last_q last_dq last_count last_time
if isempty(last_count), last_q=zeros(7,1); last_dq=zeros(7,1); last_count=0.0; last_time=-1.0e6; end
if is_new
    np=numel(position); nv=numel(velocity); last_q=zeros(7,1); last_dq=zeros(7,1);
    for k=1:min(np,7), last_q(k)=position(k); end
    for k=1:min(nv,7), last_dq(k)=velocity(k); end
    last_count=double(min(np,nv)); last_time=t;
end
joint_position=last_q; joint_count=last_count; joint_velocity=last_dq; joint_age=max(0.0,t-last_time);
end

== matlab function single_camera_xy_tracking_base_kf_fixed/Message Validation/Validate ==
  data: target_data input size=[3 1]; safe_valid output size=1; target_count input size=1; target_age input size=1; joint_position input size=[7 1]; joint_count input size=1; joint_velocity input size=[7 1]; joint_age input size=1; u output size=1; v output size=1; joint_position_out output size=[7 1]; joint_velocity_out output size=[7 1]; target_timeout_sec parameter size=1; joint_state_timeout_sec parameter size=1
function [safe_valid,u,v,joint_position_out,joint_velocity_out] = fcn(target_data,target_count,target_age,joint_position,joint_count,joint_velocity,joint_age, target_timeout_sec, joint_state_timeout_sec)
%#codegen
u=0.0; v=0.0; joint_position_out=zeros(7,1); joint_velocity_out=zeros(7,1);
target_ok=target_count>=3 && target_data(1)>0.5 && isfinite(target_data(2)) && isfinite(target_data(3)) && isfinite(target_age) && target_age<=target_timeout_sec;
joint_ok=joint_count>=7 && all(isfinite(joint_position(:))) && all(isfinite(joint_velocity(:))) && isfinite(joint_age) && joint_age<=joint_state_timeout_sec;
if target_ok, u=target_data(2); v=target_data(3); end
if joint_ok, joint_position_out=joint_position; joint_velocity_out=joint_velocity; end
safe_valid=target_ok && joint_ok;
end

== matlab function single_camera_xy_tracking_base_kf_fixed/Normalized Image Coordinates/Normalize ==
  data: u input size=1; e output size=[2 1]; v input size=1; z_meas output size=[2 1]; fx parameter size=1; fy parameter size=1; cx parameter size=1; cy parameter size=1; Z_hat parameter size=1
function [e,z_meas] = fcn(u,v, fx, fy, cx, cy, Z_hat)
%#codegen
ex=(u-cx)/fx; ey=(v-cy)/fy;
e=[ex;ey]; z_meas=Z_hat*e;
end
